simulink model "conventional_buck_COT"  (R2022b)
settings: Solver=ode23t  StartTime=0.0  StopTime=Tsim  MaxStep=Tstep_max  RelTol=RelTol
values from neighbouring files (symbols this model uses):
  C = 200e-6    (= 0.0002)    [conventional_buck_COT_params.m]
  CMC_en = 1    [conventional_buck_COT_params.m]
  COT_minOffTime = Tsw / 20    (= 1e-07)    [conventional_buck_COT_params.m]
  COT_onTime = Tsw * D    (= 1.66666666667e-07)    [conventional_buck_COT_params.m]
  DCM_en = 1    [conventional_buck_COT_params.m]
  I_L_int = 0.5    [conventional_buck_COT_params.m]    (also in conventional_buck_COT_sim.m = out4.simout.signals.values(end, 1))
  Kd = 0    [conventional_buck_COT_params.m]
  Ki = 25e3    (= 25000)    [conventional_buck_COT_params.m]
  Kp = 400    [conventional_buck_COT_params.m]
  L = 0.5e-6    (= 5e-07)    [conventional_buck_COT_params.m]
  R = 1    [conventional_buck_COT_params.m]    (also in conventional_buck_COT_sim.m = 50)
  r_C = 3e-3    (= 0.003)    [conventional_buck_COT_params.m]
  r_D = 5e-3    (= 0.005)    [conventional_buck_COT_params.m]
  r_dson_top = 5e-3    (= 0.005)    [conventional_buck_COT_params.m]
  r_L = 5e-3    (= 0.005)    [conventional_buck_COT_params.m]
  V_C_int = 1.0    (= 1)    [conventional_buck_COT_params.m]    (also in conventional_buck_COT_sim.m = out4.simout.signals.values(end, 3))
  v_D = 0.55    [conventional_buck_COT_params.m]
  Vin = 12    [conventional_buck_COT_params.m]    (also in conventional_buck_COT_sim.m = 5)
  Vref = 1    [conventional_buck_COT_params.m]    (also in conventional_buck_COT_sim.m = 1.2)
libraries: simulink x1, simulink_extras x1, slpidlib x1
settings Model: Creator=mluser  LastModifiedBy=mluser

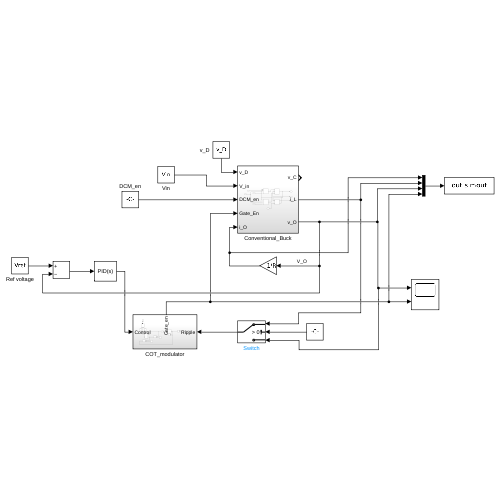
[thumbnail: Simulink's stored preview of the top-level diagram]
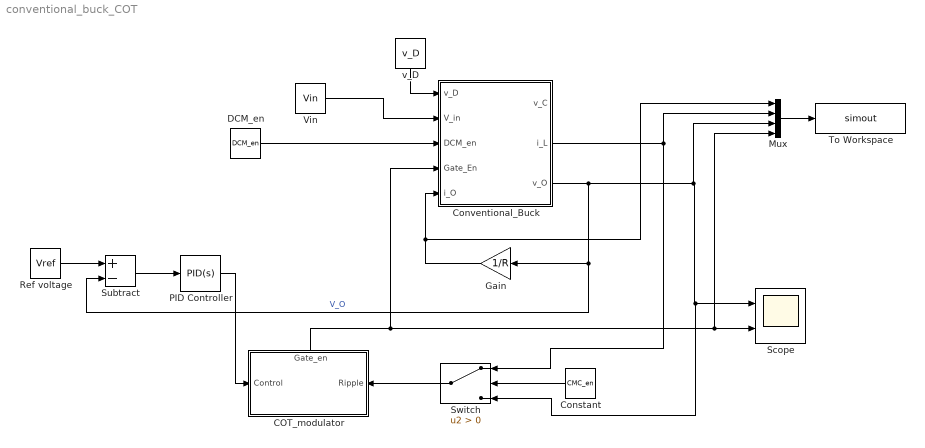
== system conventional_buck_COT ==
  COT_modulator : Subsystem
      settings: PortSchema="{\"entries\":[{\"content\":{\"sides\":[{\"content\":{\"connectorIds\":[\"In1\"]},\"type\":\"ConnectorPlacement.EquallySpacedRectSide\",\"uuid\":\"9ac7bde2-7f7d-4cc1-8d95-af26a88ce256\"},{\"content\":{\"connectorIds\":[\"In2\"],\"side\":\"RIGHT\"},\"type\":\"ConnectorPlacement.EquallySpacedRectSide\",\"uuid\":\"fdcfee6a-682f-4e93-88a2-6f56cbf72930\"},{\"content\":{\"connectorIds\":[\"Out1\"],\"side\":\"TOP\"},\"type\":\"ConnectorPlacement.EquallySpacedRectSide\",\"uuid\":\"f850504f-ff15-4b07-96e5-e684662745b4\"}]},\"type\":\"ConnectorPlacement.EquallySpacedConnector\",\"uuid\":\"a27f9dd9-b1fd-414d-b47c-912a1496f68f\"}],\"packageUris\":[\"http://schema.mathworks.com/mf0/Connector/R2020b\"],\"version\":\"1.0\"}"
  Constant : Constant  Value=CMC_en
  Conventional_Buck : Subsystem
  DCM_en : Constant  Value=DCM_en
  Gain : Gain  Gain=1/R
  Mux : Mux
  PID Controller : slpidlib/PID Controller  Controller=PID  Form=Parallel  TimeDomain=Continuous-time  UseExternalTs=off  SampleTime=-1  IntegratorMethod=Forward Euler  FilterMethod=Forward Euler  ControllerParametersSource=internal  P=Kp  I=Ki  UseKiTs=off  D=Kd  N=100  UseFilter=on  TunerSelectOption=Transfer Function Based (PID Tuner App)  InitialConditionSource=internal  InitialConditionForIntegrator=0  InitialConditionForFilter=0  DifferentiatorICPrevScaledInput=0  ExternalReset=none  TrackingMode=off  Kt=1  LimitOutput=off  SatLimitsSource=internal  UpperSaturationLimit=inf  LowerSaturationLimit=-inf  LinearizeAsGain=on  AntiWindupMode=none  Kb=1  LimitIntegrator=off  UpperIntegratorSaturationLimit=inf  LowerIntegratorSaturationLimit=-inf  POutMin=[]  POutMax=[]  IOutMin=[]  IOutMax=[]  DOutMin=[]  DOutMax=[]  NOutMin=[]  NOutMax=[]  SumOutMin=[]  SumOutMax=[]  SaturationOutMin=[]  SaturationOutMax=[]  PParamMin=[]  PParamMax=[]  IParamMin=[]  IParamMax=[]  DParamMin=[]  DParamMax=[]  NParamMin=[]  NParamMax=[]  KbParamMin=[]  KbParamMax=[]  KtParamMin=[]  KtParamMax=[]  KbOutMin=[]  KbOutMax=[]  KtOutMin=[]  KtOutMax=[]  IntegratorOutMin=[]  IntegratorOutMax=[]  FilterOutMin=[]  FilterOutMax=[]  SumI1OutMin=[]  SumI1OutMax=[]  SumI2OutMin=[]  SumI2OutMax=[]  SumI3OutMin=[]  SumI3OutMax=[]  SumI4OutMin=[]  SumI4OutMax=[]  SumDOutMin=[]  SumDOutMax=[]  DifferentiatorOutMin=[]  DifferentiatorOutMax=[]  FilterDiffOutCoefMin=[]  FilterDiffOutCoefMax=[]  ReciprocalOutMin=[]  ReciprocalOutMax=[]  SumDenOutMin=[]  SumDenOutMax=[]  SumNumOutMin=[]  SumNumOutMax=[]  DivideOutMin=[]  DivideOutMax=[]  UdiffTsProdOutMin=[]  UdiffTsProdOutMax=[]  NTsProdOutMin=[]  NTsProdOutMax=[]  UintegralTsProdOutMin=[]  UintegralTsProdOutMax=[]  UngainTsProdOutMin=[]  UngainTsProdOutMax=[]  ClampingZeroOutDataTypeStr=Inherit: Inherit via back propagation  ClampingZeroOutMin=[]  ClampingZeroOutMax=[]  FilterDenConstantOutDataTypeStr=Inherit: Inherit via back propagation  FilterDenConstantOutMin=[]  FilterDenConstantOutMax=[]  PCopyOutDataTypeStr=Inherit: Inherit via back propagation  PCopyOutMin=[]  PCopyOutMax=[]  NCopyOutDataTypeStr=Inherit: Inherit via back propagation  NCopyOutMin=[]  NCopyOutMax=[]  IntegratorContinuousStateAttributes=''  IntegratorStateMustResolveToSignalObject=off  IntegratorRTWStateStorageClass=Auto  FilterContinuousStateAttributes=''  FilterStateMustResolveToSignalObject=off  FilterRTWStateStorageClass=Auto  ParallelPVariant=InternalParameters  IdealPVariant=Disabled  IVariant=InternalParameters  DVariant=InternalParameters  IntegratorVariant=Continuous  SatVariant=Disabled  AWVariant=Passthrough  PCopyVariant=Disabled  TRVariant=Disabled  FdbkBlocksVariant=Forward  IdealPFdbkVariant=Disabled  SatFdbkVariant=Disabled  DerivativeFilterVariant=ContFilter  NVariant=InternalParameters  NCopyVariant=Disabled  FilterICVariant=InternalICsFilter  IntegratorICVariant=InternalICs  ExternalResetVariant=Disabled  TRSumVariant=Passthrough  SumFdbkVariant=Disabled  SumVariant=Sum_PID  TsampFilterVariant=InternalTs  TsampNgainVariant=Passthrough  TsampIntegralVariant=Passthrough  ExternalSaturationOutDataTypeStr=Inherit: Same as second input
  Ref voltage : Constant  Value=Vref
  Scope : Scope  NumInputPorts=2
  Subtract : Sum  Inputs=+-
  Switch : Switch  Criteria=u2 > Threshold  SaturateOnIntegerOverflow=off  InputSameDT=off
  To Workspace : ToWorkspace  VariableName=simout  SaveFormat=Structure With Time  SampleTime=-1
  Vin : Constant  Value=Vin
  v_D : Constant  Value=v_D
  wires:
  Mux/1 -> To Workspace/1
  Conventional_Buck/3(v_O) -> Mux/3, Switch/3, Scope/1, Gain/1, Subtract/2  "V_O"
  v_D/1 -> Conventional_Buck/1(v_D)
  Vin/1 -> Conventional_Buck/2(V_in)
  DCM_en/1 -> Conventional_Buck/3(DCM_en)
  Gain/1 -> Mux/1, Conventional_Buck/5(i_O)
  COT_modulator/1(Gate_en) -> Mux/4, Scope/2, Conventional_Buck/4(Gate_En)
  Conventional_Buck/2(i_L) -> Switch/1, Mux/2
  Ref voltage/1 -> Subtract/1
  Subtract/1 -> PID Controller/1
  PID Controller/1 -> COT_modulator/1(Control)
  Switch/1 -> COT_modulator/2(Ripple)
  Constant/1 -> Switch/2

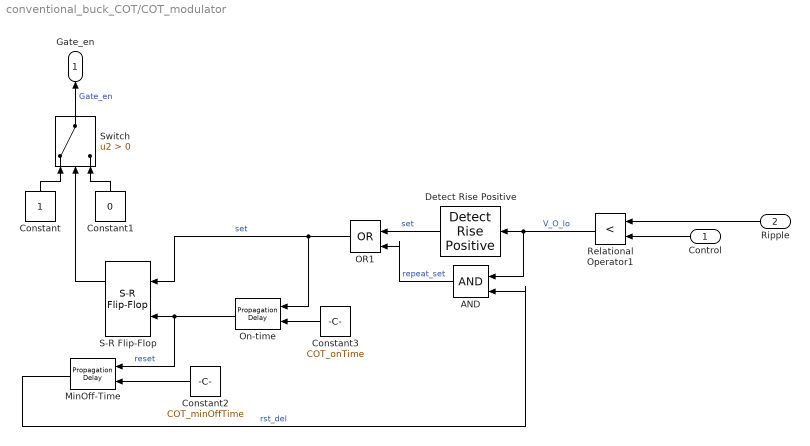
== system conventional_buck_COT/COT_modulator ==
  Control : Inport
  Ripple : Inport  Port=2
  AND : Logic  IconShape=distinctive  AllPortsSameDT=off  OutDataTypeStr=boolean
  Constant : Constant
  Constant1 : Constant  Value=0
  Constant2 : Constant  Value=COT_minOffTime
  Constant3 : Constant  Value=COT_onTime
  Detect Rise Positive : simulink/Logic and Bit Operations/Detect Rise Positive  vinit=0  OutDataTypeStr=boolean
  MinOff-Time : PropagationDelay
  OR1 : Logic  Operator=OR  IconShape=distinctive  AllPortsSameDT=off  OutDataTypeStr=boolean
  On-time : PropagationDelay
  Relational Operator1 : RelationalOperator  Operator=<  OutDataTypeStr=boolean  RndMeth=Simplest  InputSameDT=off
  S-R Flip-Flop : simulink_extras/Flip Flops/S-R Flip-Flop  initial_condition=0
  Switch : Switch  Criteria=u2 > Threshold  SaturateOnIntegerOverflow=off  InputSameDT=off
  Gate_en : Outport
  wires:
  Constant1/1 -> Switch/3
  Switch/1 -> Gate_en/1  "Gate_en"
  Control/1 -> Relational Operator1/2
  S-R Flip-Flop/1 -> Switch/2
  AND/1 -> OR1/2  "repeat_set"
  On-time/1 -> MinOff-Time/1, S-R Flip-Flop/2  "reset"
  MinOff-Time/1 -> AND/2  "rst_del"
  Detect Rise Positive/1 -> OR1/1  "set"
  Constant/1 -> Switch/1
  Constant3/1 -> On-time/2
  Constant2/1 -> MinOff-Time/2
  Ripple/1 -> Relational Operator1/1
  OR1/1 -> On-time/1, S-R Flip-Flop/1  "set"
  Relational Operator1/1 -> AND/1, Detect Rise Positive/1  "V_O_lo"

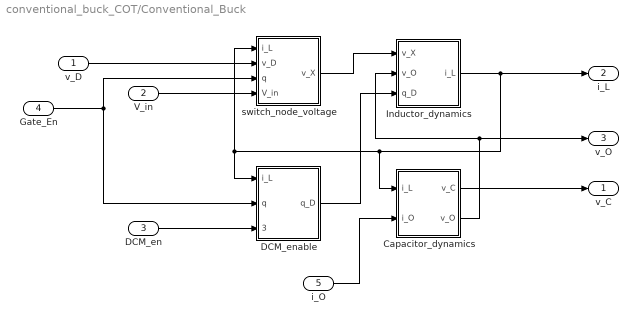
== system conventional_buck_COT/Conventional_Buck ==
  v_D : Inport
  V_in : Inport  Port=2
  DCM_en : Inport  Port=3
  Gate_En : Inport  Port=4
  i_O : Inport  Port=5
  Capacitor_dynamics : Subsystem
  DCM_enable : Subsystem
  Inductor_dynamics : Subsystem
  switch_node_voltage : Subsystem
  v_C : Outport
  i_L : Outport  Port=2
  v_O : Outport  Port=3
  wires:
  switch_node_voltage/1(v_X) -> Inductor_dynamics/1(v_X)
  DCM_enable/1(q_D) -> Inductor_dynamics/3(q_D)
  v_D/1 -> switch_node_voltage/2(v_D)
  Capacitor_dynamics/2(v_O) -> v_O/1, Inductor_dynamics/2(v_O)
  Capacitor_dynamics/1(v_C) -> v_C/1
  V_in/1 -> switch_node_voltage/4(V_in)
  Gate_En/1 -> DCM_enable/2(q), switch_node_voltage/3(q)
  Inductor_dynamics/1(i_L) -> switch_node_voltage/1(i_L), DCM_enable/1(i_L), Capacitor_dynamics/1(i_L), i_L/1
  DCM_en/1 -> DCM_enable/3(DCM_enable)
  i_O/1 -> Capacitor_dynamics/2(i_O)

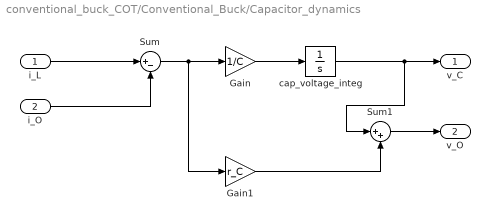
== system conventional_buck_COT/Conventional_Buck/Capacitor_dynamics ==
  i_L : Inport
  i_O : Inport  Port=2
  Gain : Gain  Gain=1/C
  Gain1 : Gain  Gain=r_C
  Sum : Sum  Inputs=|+-
  Sum1 : Sum  Inputs=|++
  cap_voltage_integ : Integrator  InitialCondition=V_C_int
  v_C : Outport
  v_O : Outport  Port=2
  wires:
  cap_voltage_integ/1 -> Sum1/1, v_C/1
  Gain/1 -> cap_voltage_integ/1
  Sum/1 -> Gain1/1, Gain/1
  i_L/1 -> Sum/1
  i_O/1 -> Sum/2
  Gain1/1 -> Sum1/2
  Sum1/1 -> v_O/1

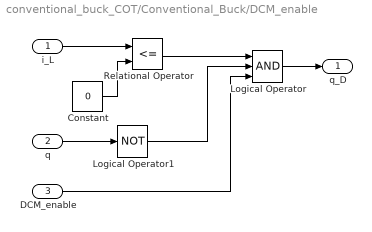
== system conventional_buck_COT/Conventional_Buck/DCM_enable ==
  i_L : Inport
  q : Inport  Port=2
  DCM_enable : Inport  Port=3
  Constant : Constant  Value=0
  Logical Operator : Logic  Inputs=3  AllPortsSameDT=off  OutDataTypeStr=boolean
  Logical Operator1 : Logic  Operator=NOT  AllPortsSameDT=off  OutDataTypeStr=boolean
  Relational Operator : RelationalOperator  Operator=<=  OutDataTypeStr=boolean  RndMeth=Simplest  InputSameDT=off
  q_D : Outport
  wires:
  i_L/1 -> Relational Operator/1
  Constant/1 -> Relational Operator/2
  Relational Operator/1 -> Logical Operator/1
  q/1 -> Logical Operator1/1
  Logical Operator1/1 -> Logical Operator/2
  DCM_enable/1 -> Logical Operator/3
  Logical Operator/1 -> q_D/1

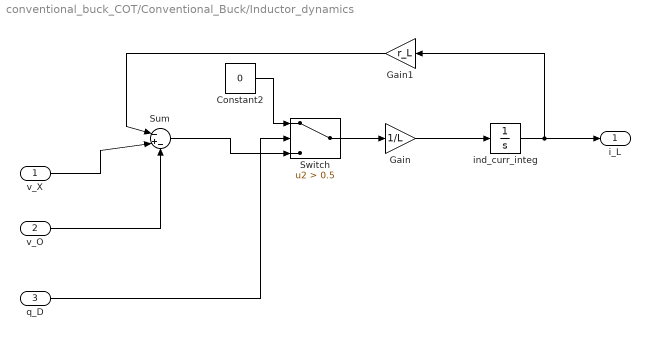
== system conventional_buck_COT/Conventional_Buck/Inductor_dynamics ==
  v_X : Inport
  v_O : Inport  Port=2
  q_D : Inport  Port=3
  Constant2 : Constant  Value=0
  Gain : Gain  Gain=1/L
  Gain1 : Gain  Gain=r_L
  Sum : Sum  Inputs=|-+-
  Switch : Switch  Criteria=u2 > Threshold  Threshold=0.5  SaturateOnIntegerOverflow=off  InputSameDT=off
  ind_curr_integ : Integrator  InitialCondition=I_L_int
  i_L : Outport
  wires:
  Constant2/1 -> Switch/1
  Gain1/1 -> Sum/1
  Sum/1 -> Switch/3
  v_O/1 -> Sum/3
  ind_curr_integ/1 -> i_L/1, Gain1/1
  Switch/1 -> Gain/1
  Gain/1 -> ind_curr_integ/1
  q_D/1 -> Switch/2
  v_X/1 -> Sum/2

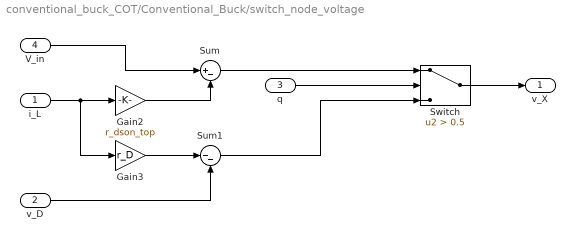
== system conventional_buck_COT/Conventional_Buck/switch_node_voltage ==
  i_L : Inport
  v_D : Inport  Port=2
  q : Inport  Port=3
  V_in : Inport  Port=4
  Gain2 : Gain  Gain=r_dson_top
  Gain3 : Gain  Gain=r_D
  Sum : Sum  Inputs=|+-
  Sum1 : Sum  Inputs=|--
  Switch : Switch  Criteria=u2 > Threshold  Threshold=0.5  SaturateOnIntegerOverflow=off  InputSameDT=off
  v_X : Outport
  wires:
  i_L/1 -> Gain3/1, Gain2/1
  V_in/1 -> Sum/1
  Gain2/1 -> Sum/2
  Sum/1 -> Switch/1
  v_D/1 -> Sum1/2
  Gain3/1 -> Sum1/1
  Sum1/1 -> Switch/3
  q/1 -> Switch/2
  Switch/1 -> v_X/1
